simulink model "PowerSystem1"  (R2017b)
settings: Solver=FixedStepAuto  StartTime=0.0  StopTime=2  FixedStep=0.0001  RelTol=1e-3
libraries: pe_lib x6, nesl_utility x3, fl_lib x2, pePowerMeasurement x1
settings Model: Creator=wai1  LastModifiedBy=wai1

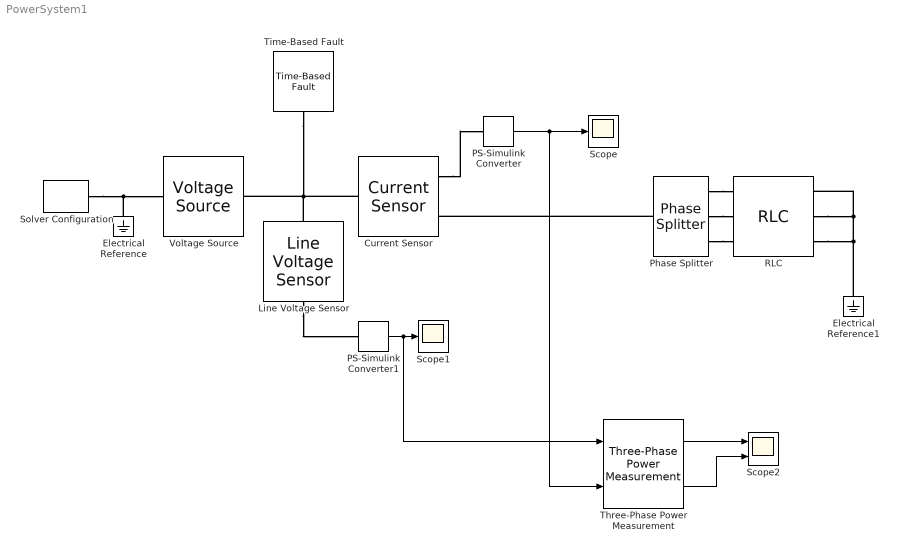
== system PowerSystem1 ==
  Current Sensor : pe_lib/Sensors/Current Sensor
      settings: SourceProductName=Simscape Power Systems  SourceProductBaseCode=PS
  Electrical Reference : fl_lib/Electrical/Electrical Elements/Electrical Reference
  Electrical Reference1 : fl_lib/Electrical/Electrical Elements/Electrical Reference
  Line Voltage Sensor : pe_lib/Sensors/Line Voltage Sensor
      settings: SourceProductName=Simscape Power Systems  SourceProductBaseCode=PS
  PS-Simulink Converter : nesl_utility/PS-Simulink Converter  PhysicalDomain=network_engine_domain  SubClassName=ps_output  LeftPortType=input  RightPortType=output  PseudoPeriodic=off  Frequencies=[]  Unit=A  AffineConversion=off
  PS-Simulink Converter1 : nesl_utility/PS-Simulink Converter  PhysicalDomain=network_engine_domain  SubClassName=ps_output  LeftPortType=input  RightPortType=output  PseudoPeriodic=off  Frequencies=[]  Unit=V  AffineConversion=off
  Phase Splitter : pe_lib/Connections/Phase Splitter
      settings: SourceProductName=Simscape Power Systems  SourceProductBaseCode=PS
  RLC : pe_lib/Passive Devices/RLC  component_structure=1  R=10 Ohm  L=1e-3 H  IL0=[0, 0, 0] A  C=1e-6 F  VC0=[0, 0, 0] V  R_parasitic=1e-6 Ohm  G_parasitic=1e-6 1/Ohm
      settings: SourceProductName=Simscape Power Systems  SourceProductBaseCode=PS
  Scope : Scope
  Scope1 : Scope
  Scope2 : Scope  NumInputPorts=2
  Solver Configuration : nesl_utility/Solver Configuration  PhysicalDomain=network_engine_domain  SubClassName=solver  LeftPortType=input  RightPortType=generic  Accelerate=off  Tones=[]  Harmonics=[]  SimulateNoise=off  Profile=off  UseLocalSampling=off  EnableSwitchedLinearOptims=on  FrequencyDomain=off  UseCCode=off  RelTol=0.001  AbsTol=1e-06  MinStep=1e-09  ToWorkspace=off  RevertToSquareIcSolve=off  NumHomotopyIterations=100  PhasorMode=off  PhasorModeNumHarmonics=1  DoDC=off  ResidualTolerance=1e-09  UseLocalSolver=off  LocalSolverChoice=NE_BACKWARD_EULER_ADVANCER  LocalSolverSampleTime=0.001  DoFixedCost=off  MaxNonlinIter=3  MaxModeIter=2  LinearAlgebra=Sparse  DelaysMemoryBudget=1024  AutomaticFiltering=on  FilteringTimeConstant=0.001
  Three-Phase Power Measurement : pePowerMeasurement/Three-Phase Power Measurement  OverrideUsingVariant=Continuous  F=60  K=[0 1 2 3]  Seq=Positive  Ts=0
  Time-Based Fault : pe_lib/Passive Devices/Faults/Time-Based Fault  fault_type_option=7  R_pn_fault=1e-3 Ohm  R_ng_fault=1e-3 Ohm  G_parasitic=1e-6 1/Ohm  fault_start_time=1 s  fault_duration=0.3 s  R_pn_nofault=1e6 Ohm  G_ng_fault=1e3 1/Ohm  fault_stop_time=0 s
      settings: SourceProductName=Simscape Power Systems  SourceProductBaseCode=PS
  Voltage Source : pe_lib/Sources/Voltage Source  vline_rms=sqrt(3) * 100 / sqrt(2) V  shift=0 deg  freq=60 Hz  impedance_option=1  SShortCircuit=1e6 V*A  XR=15  R=0.01 Ohm  L=3.97e-4 H  G_parasitic=0 1/Ohm  harmonic_option=0  harmonic_orders=[5, 7, 11, 13]  harmonic_ratios=[.1, .1, .1, .1]  I_specify=off  I_priority=None  I=[ 0 0 0 ] A  I_nominal_specify=off  I_nominal_unit=A  I_nominal_value=1
      settings: SourceProductName=Simscape Power Systems  SourceProductBaseCode=PS
  wires:
  PS-Simulink Converter/1 -> Three-Phase Power Measurement/2, Scope/1
  PS-Simulink Converter1/1 -> Three-Phase Power Measurement/1, Scope1/1
  Three-Phase Power Measurement/1 -> Scope2/1
  Three-Phase Power Measurement/2 -> Scope2/2
  connections:
  Electrical Reference/LConn1 -- Solver Configuration/RConn1 -- Voltage Source/LConn1
  Current Sensor/LConn1 -- Time-Based Fault/LConn1 -- Line Voltage Sensor/LConn1 -- Voltage Source/RConn1
  Electrical Reference1/LConn1 -- RLC/RConn3 -- RLC/RConn2 -- RLC/RConn1
  Phase Splitter/LConn1 -- Current Sensor/RConn2
  Phase Splitter/RConn1 -- RLC/LConn1
  Phase Splitter/RConn2 -- RLC/LConn2
  Phase Splitter/RConn3 -- RLC/LConn3
  Current Sensor/RConn1 -- PS-Simulink Converter/LConn1
  Line Voltage Sensor/RConn1 -- PS-Simulink Converter1/LConn1
